simulink model "quadra_model"  (R2023a)
settings: Solver=FixedStepDiscrete  StartTime=0.0  StopTime=tmax  FixedStep=tstep  RelTol=1e-3
values from neighbouring files (symbols this model uses):
  a_fxd = (fi(a_dbl,dt.coeff_fxd.s,dt.coeff_fxd.w,dt.coeff_fxd.f))'    [run_main.m]
  Af = 1    [params.m]
  b_fxd = (fi(b_dbl,dt.coeff_fxd.s,dt.coeff_fxd.w,dt.coeff_fxd.f))'    [run_main.m]
  Bf = 2    [params.m]
  c_fxd = (fi(c_dbl,dt.coeff_fxd.s,dt.coeff_fxd.w,dt.coeff_fxd.f))'    [run_main.m]
  Cf = -pi/4    (= -0.785398163397)    [params.m]
  LUT_breakpoints = 0:LUT_size-1    [run_main.m]
  req_accuracy = 5.25e-6    (= 5.25e-06)    [params.m]
undefined symbols (not defined in the file or in its folder): dt
libraries: simulink x3
settings Model: DataTypeOverride=Off  Creator=szymadej  LastModifiedBy=szymadej
settings SolverCC: AlgebraicLoopSolver=TrustRegion
settings DataIOCC: LimitDataPoints=on  SaveOutput=off  SaveTime=off
settings OptimizationCC: BlockReduction=off  ConditionallyExecuteInputs=off  DefaultParameterBehavior=Inlined  ExpressionDepthLimit=2147483647  InitFltsAndDblsToZero=on  LifeSpan=inf
settings DebuggingCC: AlgebraicLoopMsg=error  UnderspecifiedInitializationDetection=Classic  MergeDetectMultiDrivingBlocksExec=none  SingleTaskRateTransMsg=error  FcnCallInpInsideContextMsg=warning  UnconnectedInputMsg=warning  UnconnectedOutputMsg=warning  UnconnectedLineMsg=warning  AllowSymbolicDim=off  StateNameClashWarn=warning  StrictBusMsg=ErrorOnBusTreatedAsVector  SFUnexpectedBacktrackingDiag=warning  SFNoUnconditionalDefaultTransitionDiag=warning  SFExecutionAtInitializationDiag=none  ArithmeticOperatorsInVariantConditions=warning
settings HardwareCC: ProdBitPerPointer=32  ProdBitPerSizeT=32  ProdBitPerPtrDiffT=32  ProdLargestAtomicFloat=None  ProdIntDivRoundTo=Undefined  ProdEndianess=Unspecified  ProdWordSize=32  ProdHWDeviceType=ASIC/FPGA->ASIC/FPGA  ProdEqTarget=off
settings ModelReferenceCC: EnableRefExpFcnMdlSchedulingChecks=on
settings SFSimCC: SimUseLocalCustomCode=off  SimParseCustomCode=off  CustomCodeUndefinedFunction=UseInterfaceOnly
settings RTWCC: RTWUseLocalCustomCode=off
settings CodeAppCC: StateflowObjectComments=on
settings GRTTargetCC: TargetLangStandard=C89/C90 (ANSI)  CombineOutputUpdateFcns=off  GRTInterface=on
settings ConfigComp: CovScope=ReferencedModels  CovMetricSettings=dw  CovSaveCumulativeToWorkspaceVar=on  CovSaveSingleToWorkspaceVar=on  CovExternalEMLEnable=off  CovSFcnEnable=off

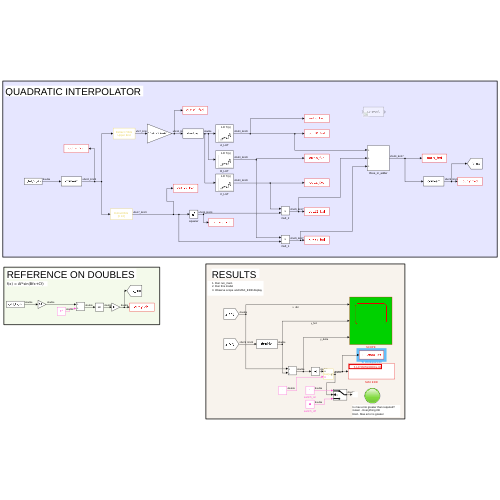
[thumbnail: Simulink's stored preview of the top-level diagram]
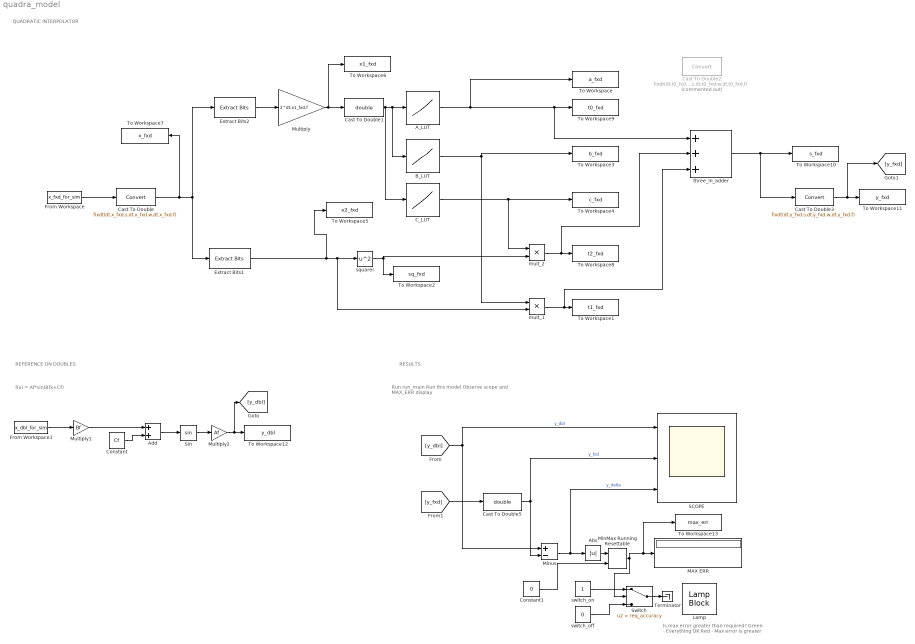
== system quadra_model ==
  note: REFERENCE ON DOUBLES
  note: QUADRATIC INTERPOLATOR
  note: RESULTS
  note: Is max error greater than required?
      | Green - Everything OK
      | Red - Max error is greater
  note: Run run_main
      | Run this model
      | Observe scope and MAX_ERR display
  note: f(x) = Af*sin(Bfx+Cf)
  A_LUT : Lookup_n-D  NumberOfTableDimensions=1  BreakpointsForDimension1=LUT_breakpoints  BreakpointsForDimension1DataTypeStr=Inherit: Inherit from 'Breakpoint data'  IndexSearchMethod=Evenly spaced points  Table=a_fxd  TableDataTypeStr=Inherit: Inherit from 'Table data'  InterpMethod=Flat  DiagnosticForOutOfRangeInput=Warning  InternalRulePriority=Speed  OutDataTypeStr=Inherit: Inherit from 'Table data'  RndMeth=Zero
  Abs : Abs  SaturateOnIntegerOverflow=off
  Add : Sum
  B_LUT : Lookup_n-D  NumberOfTableDimensions=1  BreakpointsForDimension1=LUT_breakpoints  BreakpointsForDimension1DataTypeStr=Inherit: Inherit from 'Breakpoint data'  IndexSearchMethod=Evenly spaced points  Table=b_fxd  TableDataTypeStr=Inherit: Inherit from 'Table data'  InterpMethod=Flat  DiagnosticForOutOfRangeInput=Warning  InternalRulePriority=Speed  OutDataTypeStr=Inherit: Inherit from 'Table data'  RndMeth=Simplest
  C_LUT : Lookup_n-D  NumberOfTableDimensions=1  BreakpointsForDimension1=LUT_breakpoints  BreakpointsForDimension1DataTypeStr=Inherit: Inherit from 'Breakpoint data'  IndexSearchMethod=Evenly spaced points  Table=c_fxd  TableDataTypeStr=Inherit: Inherit from 'Table data'  InterpMethod=Flat  DiagnosticForOutOfRangeInput=Warning  InternalRulePriority=Speed  OutDataTypeStr=Inherit: Inherit from 'Table data'  RndMeth=Simplest
  Cast To Double : DataTypeConversion  OutDataTypeStr=fixdt(dt.x_fxd.s,dt.x_fxd.w,dt.x_fxd.f)  SaturateOnIntegerOverflow=off  RndMeth=Floor
  Cast To Double1 : DataTypeConversion  OutDataTypeStr=double  SaturateOnIntegerOverflow=off  RndMeth=Floor
  Cast To Double2 : DataTypeConversion  Commented=on  OutDataTypeStr=fixdt(dt.t0_fxd.s,dt.t0_fxd.w,dt.t0_fxd.f)  SaturateOnIntegerOverflow=off  RndMeth=Floor
  Cast To Double3 : DataTypeConversion  OutDataTypeStr=fixdt(dt.y_fxd.s,dt.y_fxd.w,dt.y_fxd.f)  SaturateOnIntegerOverflow=off  RndMeth=Floor
  Cast To Double5 : DataTypeConversion  OutDataTypeStr=double  SaturateOnIntegerOverflow=off  RndMeth=Floor
  Constant : Constant  Value=Cf
  Constant1 : Constant  Value=0
  Extract Bits1 : simulink/Logic and Bit Operations/Extract Bits  bitsToExtract=Range of bits  numBits=17  bitIdxRange=[0 dt.x2_fxd.w-1]  outScalingMode=Preserve fixed-point scaling
  Extract Bits2 : simulink/Logic and Bit Operations/Extract Bits  bitsToExtract=Range starting with most significant bit  numBits=m  bitIdxRange=[23 17]  outScalingMode=Preserve fixed-point scaling
  From Workspace : FromWorkspace  VariableName=x_fxd_for_sim  OutDataTypeStr=double  Interpolate=off  OutputAfterFinalValue=Setting to zero
  From Workspace1 : FromWorkspace  VariableName=x_dbl_for_sim  OutDataTypeStr=double  Interpolate=off  OutputAfterFinalValue=Setting to zero
  Lamp : LampBlock  LabelPosition=Hide
  MAX ERR : Display
  MinMax Running Resettable : simulink/Math Operations/MinMax Running Resettable  Function=max  vinit=0.0
  Minus : Sum  Inputs=+-
  Multiply : Gain  Gain=2^dt.x1_fxd.f
  Multiply1 : Gain  Gain=Bf
  Multiply2 : Gain  Gain=Af
  SCOPE : Scope  NumInputPorts=3
  Sin : Trigonometry
  Switch : Switch  Criteria=u2 > Threshold  Threshold=req_accuracy  SaturateOnIntegerOverflow=off  InputSameDT=off
  Terminator : Terminator
  To Workspace : ToWorkspace  VariableName=a_fxd  SampleTime=-1
  To Workspace1 : ToWorkspace  VariableName=t1_fxd  SampleTime=-1
  To Workspace10 : ToWorkspace  VariableName=s_fxd  SampleTime=-1
  To Workspace11 : ToWorkspace  VariableName=y_fxd  SampleTime=-1
  To Workspace12 : ToWorkspace  VariableName=y_dbl  SampleTime=-1
  To Workspace13 : ToWorkspace  VariableName=max_err  SampleTime=-1
  To Workspace2 : ToWorkspace  VariableName=sq_fxd  SampleTime=-1
  To Workspace3 : ToWorkspace  VariableName=b_fxd  SampleTime=-1
  To Workspace4 : ToWorkspace  VariableName=c_fxd  SampleTime=-1
  To Workspace5 : ToWorkspace  VariableName=x2_fxd  SampleTime=-1
  To Workspace6 : ToWorkspace  VariableName=x1_fxd  SampleTime=-1
  To Workspace7 : ToWorkspace  VariableName=x_fxd  SampleTime=-1
  To Workspace8 : ToWorkspace  VariableName=t2_fxd  SampleTime=-1
  To Workspace9 : ToWorkspace  VariableName=t0_fxd  SampleTime=-1
  mult_1 : Product  OutDataTypeStr=fixdt(dt.t1_fxd.s,dt.t1_fxd.w,dt.t1_fxd.f)
  mult_2 : Product  OutDataTypeStr=fixdt(dt.t2_fxd.s,dt.t2_fxd.w,dt.t2_fxd.f)
  squarer : Math  Operator=square  OutDataTypeStr=fixdt(dt.sq_fxd.s,dt.sq_fxd.w,dt.sq_fxd.f)
  switch_off : Constant  Value=0
  switch_on : Constant
  three_in_adder : Sum  Inputs=+++  OutDataTypeStr=fixdt(dt.s_fxd.s,dt.s_fxd.w,dt.s_fxd.f)
  wires:
  From Workspace/1 -> Cast To Double/1
  Cast To Double/1 -> To Workspace7/1, Extract Bits2/1, Extract Bits1/1
  Extract Bits2/1 -> Multiply/1
  Multiply/1 -> To Workspace6/1, Cast To Double1/1
  Cast To Double1/1 -> C_LUT/1, B_LUT/1, A_LUT/1
  Extract Bits1/1 -> To Workspace5/1, mult_1/2, squarer/1
  B_LUT/1 -> To Workspace3/1, mult_1/1
  mult_1/1 -> three_in_adder/3, To Workspace1/1
  squarer/1 -> To Workspace2/1, mult_2/2
  C_LUT/1 -> To Workspace4/1, mult_2/1
  mult_2/1 -> three_in_adder/2, To Workspace8/1
  A_LUT/1 -> three_in_adder/1, To Workspace9/1, To Workspace/1
  three_in_adder/1 -> Cast To Double3/1, To Workspace10/1
  Cast To Double3/1 -> [y_fxd], To Workspace11/1
  Constant/1 -> Add/2
  From Workspace1/1 -> Multiply1/1
  Add/1 -> Sin/1
  Multiply1/1 -> Add/1
  [y_fxd] -> Cast To Double5/1
  [y_dbl] -> Minus/1, SCOPE/1  "y_dbl"
  Cast To Double5/1 -> Minus/2, SCOPE/2  "y_fxd"
  Minus/1 -> Abs/1, SCOPE/3  "y_delta"
  MinMax Running Resettable/1 -> Switch/2, To Workspace13/1, MAX ERR/1
  switch_on/1 -> Switch/1
  switch_off/1 -> Switch/3
  Switch/1 -> Terminator/1
  Abs/1 -> MinMax Running Resettable/1
  Sin/1 -> Multiply2/1
  Multiply2/1 -> [y_dbl], To Workspace12/1
  Constant1/1 -> MinMax Running Resettable/2
